simulink model "VMC_LateralTrajectoryPlanningControllerV04"  (R2018b)
settings: Solver=FixedStepDiscrete  StartTime=0.0  StopTime=10  FixedStep=0.02  RelTol=1e-3
values from neighbouring files (symbols this model uses):
  D_d_end = 0    [TRP_parameters.m]
  P_optimizer_interations = 5.0    (= 5)    [TRP_parameters.m]
  P_TRP_Lat_dT = 0.02    [TRP_parameters.m]
  P_Vehicle_width = 1.8    [TRP_parameters.m]
  P_vVeh_min_TrajCalc = 5.0    (= 5)    [TRP_parameters.m]
libraries: simulink x1
(part 2 of 2)

== matlab function VMC_LateralTrajectoryPlanningControllerV04/VMC_LateralTrajectoryPlanningController/LatTRP_GenerateTraj/MATLAB Function ==
  data: vVeh input; SafetyDistance input; B_StartOptimization input; B_StopOptimization input; d_start input; d_d_start input; d_dd_start input; d_ddd_start_K1 input; t_max_in input; t_min_in input; k_j input; k_v input; k_t input; k_cy input; k_j_y_constraint input; k_a_y_constraint input; k_overshoot input; k_jy_change_sq input; j_y_constraint input; a_y_constraint input; d_overshootAllowed input; d_left_yellow input; d_right_yellow input; d_end input; P_vVeh_min_TrajCalc parameter; P_optimizer_interations parameter; P_TRP_Lat_dT parameter; P_Vehicle_width parameter; d0 output; d1 output; d2 output; d3 output; d4 output; d5 output; s_end_traj output; c2 input; t_Winner output
function [d0, d1, d2, d3, d4, d5, s_end_traj, t_Winner] = fcn(vVeh,SafetyDistance,B_StartOptimization,B_StopOptimization,d_start,d_d_start,d_dd_start,d_ddd_start_K1,t_max_in,...
                                              t_min_in,k_j,k_v,k_t,k_cy,k_j_y_constraint,k_a_y_constraint,k_overshoot,k_jy_change_sq,j_y_constraint,a_y_constraint,...
                                              d_overshootAllowed, d_left_yellow,d_right_yellow,d_end,P_vVeh_min_TrajCalc,...
                                              P_optimizer_interations,P_TRP_Lat_dT,P_Vehicle_width, c2)
D_dT = P_TRP_Lat_dT;

persistent d0_K1;
persistent d1_K1;
persistent d2_K1;
persistent d3_K1;
persistent d4_K1;
persistent d5_K1;
persistent t_min_K1
persistent t_max_K1
persistent alreadyCalculated
persistent t
persistent d3_opt
persistent d4_opt
persistent d5_opt
persistent a_y_violation
persistent j_y_violation
persistent jerk_sq_int
persistent jy_change_sq
persistent vel_sq_int
persistent cost
persistent violation_sq_left_yellow_int
persistent violation_sq_right_yellow_int
persistent d_overshoot_violation
persistent s_end_traj_
persistent winner

if isempty(d0_K1)
    d0_K1 = 0;
    d1_K1 = 0;
    d2_K1 = 0;
    d3_K1 = 0;
    d4_K1 = 0;
    d5_K1 = 0;
    t_min_K1 = 0;
    t_max_K1 = 0;
    alreadyCalculated = false(5,1);
    t = zeros(5,1);
    d3_opt = zeros(5,1);
    d4_opt = zeros(5,1);
    d5_opt = zeros(5,1);
    a_y_violation = zeros(5,1);
    j_y_violation = zeros(5,1);
    jerk_sq_int = zeros(5,1);
    jy_change_sq = zeros(5,1);
    vel_sq_int = zeros(5,1);
    cost = zeros(5,1);
    violation_sq_left_yellow_int = zeros(5,1);
    violation_sq_right_yellow_int = zeros(5,1);
    d_overshoot_violation = zeros(5,1);
    s_end_traj_ = 0;
    winner = 1;
end

% fisrt three coefficients are independent of the trajecotry length
d0_opt = d_start;
d1_opt = d_d_start;
d1_opt_p2 = d1_opt * d1_opt;
d2_opt = 0.5 * d_dd_start;
d2_opt_p2 = d2_opt * d2_opt;

% start values for the duration for the optimization
% if B_startoptimization flag is true, new trajectory optimization starts
% get the initial trajectory length limits from input arguments;

if B_StartOptimization == true
    t_min = t_min_in;
    t_max = t_max_in;
    
    alreadyCalculated(1) = false;
    alreadyCalculated(2) = false;
    alreadyCalculated(3) = false;
    alreadyCalculated(4) = false;
    alreadyCalculated(5) = false;
% otherwise, set the trajectory length limits according to the best
% trajectory from previous cycle
else
    t_min = t_min_K1;
    t_max = t_max_K1;
end

% limit velocity to prevent short and vary dynamic trajecotry at low
% velocity
vVeh_lim = vVeh;
vVeh_lim = max(vVeh_lim,P_vVeh_min_TrajCalc);
vVeh_lim_p2 = vVeh_lim * vVeh_lim;
vVeh_lim_p4 = vVeh_lim_p2 * vVeh_lim_p2;
vVeh_lim_p6 = vVeh_lim_p4 * vVeh_lim_p2;

% if both B_startoptimization B_stopoptimization flags are true
% it indicates all the optimization interations will be done in one
% calculation cycle

if B_StartOptimization == true && B_StopOptimization == true
    
    OptimizerInterations = P_optimizer_interations;
    % otherwise only one optimization interation will run during each
    % calculation cycle
else
    OptimizerInterations = 1;
end

for index = 1:OptimizerInterations
    % divide interval
    delta_t = (t_max - t_min) / 4;
    t(1) = t_min;
    t(2) = t_min + delta_t;
    t(3) = t_min + 2 * delta_t;
    t(4) = t_min + 3 * delta_t;
    t(5) = t_max;
    
    for i = 1:5
        i_lim = min(i,5);
        % only calculate and evaluate the trajectory if it has not already
        % been calculated and evaluated in the previous iteration
        % short and dynamic trajectories at low speed
        if ~alreadyCalculated(i_lim)
            s_end = t(i_lim) * vVeh_lim;
            s_end_p2 = s_end * s_end;
            s_end_p3 = s_end_p2 * s_end;
            s_end_p4 = s_end_p3 * s_end;
            s_end_p5 = s_end_p4 * s_end;
            s_end_p6 = s_end_p5 * s_end;
            s_end_p7 = s_end_p6 * s_end;
            s_end_p8 = s_end_p7 * s_end;
            s_end_p9 = s_end_p8 * s_end;
            
             % calculate remaining coefficient;
            d3_opt(i_lim) = -(3 * d_dd_start * s_end_p2 + 12  * d_d_start * s_end - 20 * d_end + 20 * d_start) / (2 * s_end_p3);
            d3_opt_p2 = d3_opt(i_lim) * d3_opt(i_lim);
            d4_opt(i_lim) = (3 * d_dd_start * s_end_p2 + 16 * d_d_start * s_end - 30 * d_end + 30 * d_start) / (2 * s_end_p4);
            d4_opt_p2 = d4_opt(i_lim) * d4_opt(i_lim);
            d5_opt(i_lim) = -(d_dd_start * s_end_p2 + 6 * d_d_start * s_end - 12 * d_end + 12 * d_start) / (2 * s_end_p5);
            d5_opt_p2 = d5_opt(i_lim) * d5_opt(i_lim);
            
            % calculate points on trajectory with max kappa if d5 is not
            % too close to 0 (division by 0)
            
            if abs(d5_opt(i_lim)) > 1e-20
                s_kappa_max_temp = (2 * d4_opt(i_lim)) / (10 * d5_opt(i_lim)) * (2 * d4_opt(i_lim)) / (10 * d5_opt(i_lim)) - d3_opt(i_lim) / (10 * d5_opt(i_lim));
                s_kappa_max_temp = sqrt(s_kappa_max_temp);
                s_kappa_max_1 = -(2 * d4_opt(i_lim)) / (10 * d5_opt(i_lim)) - s_kappa_max_temp;
                s_kappa_max_1 = max(0,s_kappa_max_1);
                s_kappa_max_1 = min(s_kappa_max_1,s_end);
                s_kappa_max_2 = -(2 * d4_opt(i_lim)) / (10 * d5_opt(i_lim)) + s_kappa_max_temp;
                s_kappa_max_2 = max(s_kappa_max_2,0);
                s_kappa_max_2 = min(s_kappa_max_2,s_end);
                
                
                s_kappa_max_1_p2 = s_kappa_max_1 * s_kappa_max_1;
                s_kappa_max_1_p3 = s_kappa_max_1_p2 * s_kappa_max_1;
                
                s_kappa_max_2_p2 = s_kappa_max_2 * s_kappa_max_2;
                s_kappa_max_2_p3 = s_kappa_max_2_p2 * s_kappa_max_2;
            else
                % if d5 is too close to 0 then set the position to -1 
                % this will lead to neglecting the maximum lateral
                % acceleratio in the cost function
                % s_kappa_max_temp = -1;
                s_kappa_max_1 = -1;
                s_kappa_max_2 = -1;
                
                s_kappa_max_1_p2 = -1;
                s_kappa_max_1_p3 = -1;
                
                s_kappa_max_2_p2 = -1;
                s_kappa_max_2_p3 = -1;
                
                 % Idea: if d5 is chose to 0,then calculate max lateral acceleration with polynomial of degree 4 if possible
            end
            
            % calculate max lateral acceleration under the assumption of constant curvature and vehicle velocity. but only if the
            % point at a relevant position(>= 0 and <= planned length s_end)
            
            if (s_kappa_max_1 >= 0 && s_kappa_max_1 <= s_end)
                a_y_1_abs = vVeh * vVeh * c2 + vVeh * vVeh * (2 * d2_opt + 6 * d3_opt(i_lim) * s_kappa_max_1 + 12 * d4_opt(i_lim) * s_kappa_max_1_p2 + 20 * d5_opt(i_lim) * s_kappa_max_1_p3);
                a_y_1_abs = abs(a_y_1_abs);
            else
                a_y_1_abs = 0;
            end
            
            if (s_kappa_max_2 >= 0 && s_kappa_max_2 <= s_end)
                a_y_2_abs = vVeh * vVeh * c2 + vVeh * vVeh * (2 * d2_opt + 6 * d3_opt(i_lim) * s_kappa_max_2 + 12 * d4_opt(i_lim) * s_kappa_max_2_p2 + 20 * d5_opt(i_lim) * s_kappa_max_2_p3);
                a_y_2_abs = abs(a_y_2_abs);
            else
                a_y_2_abs = 0;
            end
            % find maximum acceleration value
            % start and end is not considered because they are both boundary conditions
            a_abs_max = a_y_1_abs;
            a_abs_max = max(a_abs_max,a_y_2_abs);
            a_y_violation(i_lim) = a_abs_max - a_y_constraint;
            a_y_violation(i_lim) = max(a_y_violation(i_lim),0);
            
             % find max jerk in trajectory under the assumption: the
            % reference line has no jerk itself (constant curvature)
            % find position of extremum and calculate the jerk at this position
            if abs(d5_opt(i_lim)) > 1e-20
                s_jerk_max = -24 * d4_opt(i_lim) / (120 * d5_opt(i_lim));
                
                % limit position to trajectory length
                s_jerk_max = max(s_jerk_max,0);
                s_jerk_max = min(s_jerk_max,s_end);
                
                % calculate lateral jerk at extremum
                j_y_l_abs = vVeh * vVeh * vVeh * (6 * d3_opt(i_lim) + 24 * d4_opt(i_lim) * s_jerk_max + 60 * d5_opt(i_lim) * s_jerk_max * s_jerk_max);
                j_y_l_abs = abs(j_y_l_abs);
            else
                % if d5 is 0 then the jerk is linear, therefore the
                % absolute maximum of the lateral jerk of the trajectory
                % has to occur at the position 0 and s_end (they are
                % covered by j_y_2_abs and j_y_3_abs)
                % s_jerk_max = 0;
                j_y_l_abs = 0;
            end
            % calculate lateral jerk at the start and at the end of the
            % trajectory
            j_y_2_abs = vVeh * vVeh * vVeh * (6 * d3_opt(i_lim) + 24 * d4_opt(i_lim) * s_end + 60 * d5_opt(i_lim) * s_end_p2);
            j_y_2_abs = abs(j_y_2_abs);
            j_y_3_abs = vVeh * vVeh * vVeh * 6 * d3_opt(i_lim);
            j_y_3_abs = abs(j_y_3_abs);
            j_abs_max = j_y_l_abs;
            j_abs_max = max(j_abs_max,j_y_2_abs);
            j_abs_max = max(j_abs_max,j_y_3_abs);
            
            j_y_violation(i_lim) = j_abs_max - j_y_constraint;
            j_y_violation(i_lim) = max(j_y_violation(i_lim),0);
            
             % calculate the integral of jerk squared
            jerk_sq_int(i_lim) = (12 * s_end * vVeh_lim_p6 * (3 * d3_opt_p2 + 12 * d3_opt(i_lim) * d4_opt(i_lim) * s_end + 20 * d3_opt(i_lim) * d5_opt(i_lim) * s_end_p2 + 16 * d4_opt_p2 * s_end_p2 + 60 * d4_opt(i_lim) * d5_opt(i_lim) * s_end_p3 + 60 * d5_opt_p2 * s_end_p4)) / vVeh_lim;
            
            % calculate the change in lateral jerk squared at the beginning
            % of the trajectory(compared to the lateral jerk at the
            % beginning of the last trajectory)
            jy_change_sq(i_lim) = vVeh * vVeh * vVeh * (6 * d3_opt(i_lim) - d_ddd_start_K1);
            jy_change_sq(i_lim) = jy_change_sq(i_lim) * jy_change_sq(i_lim);
            
            % calculate the integral of acceleration squared
            % accel_sq_int = (4 *d2_p2 * s_end * vVeh_lim_p4 + (s_end_p3 * vVeh_lim_p4 *(36 * d3_opt_p2 + 48 * d2 *d4_opt(i_lim))/3 +  (s_end_p5 * vVeh_lim_p4 * (144 * d4_opt_p2 + 240 * d3_opt(i_lim) * d5_opt(i_lim)) / 5 + (s_end_p4 * vVeh_lim_p4 * (80 * d2 * d5_opt(i_lim) + 144 * d4_opt(i_lim) * d4_opt(i_lim)) / 4 + (400 * d5_opt_p2 * s_end_p7 * vVeh_lim_p4) / 7 + 12 * d2 * d3_opt(i_lim) * s_end_p2 * vVeh_lim_p4 + 80 * d4_opt(i_lim) * d5_opt(i_lim) * s_end_p6 * vVeh_lim_p4) / vVeh_lim;
            
            % calculate the integral of velocity squared
            vel_sq_int(i_lim) = (d1_opt_p2 * s_end * vVeh_lim_p2 + (s_end_p3 * vVeh_lim_p2 * (4 * d2_opt_p2 + 6 * d1_opt * d3_opt(i_lim))) / 3 + (s_end_p7 * vVeh_lim_p2 * (16 * d4_opt_p2 + 30 * d3_opt(i_lim) * d5_opt(i_lim))) / 7 + (s_end_p4 * vVeh_lim_p2 * (8 * d1_opt * d4_opt(i_lim) + 12 * d2_opt * d3_opt(i_lim))) / 4 + (s_end_p6 * vVeh_lim_p2 * (20 * d2_opt * d5_opt(i_lim)+ 24 * d3_opt(i_lim) * d4_opt(i_lim))) / 6 + (25 * d5_opt_p2 * s_end_p9 * vVeh_lim_p2) / 9 + (s_end_p5 * vVeh_lim_p2 * (9 * d3_opt_p2 + 10 * d1_opt * d5_opt(i_lim) + 16 * d2_opt * d4_opt(i_lim))) / 5 + 2 * d1_opt * d2_opt * s_end_p2 * vVeh_lim_p2 + 5 * d4_opt(i_lim) * d5_opt(i_lim) * s_end_p8 * vVeh_lim_p2) / vVeh_lim;
            
             % calculate the space of violation of left yellow corridor border
            [violationAreaLeft,violationAreaRight] = LatCorridorViolationCheck(P_Vehicle_width,SafetyDistance,d0_opt,d1_opt,d2_opt,d3_opt(i_lim),d4_opt(i_lim),d5_opt(i_lim),s_end,d_left_yellow,d_right_yellow,vVeh_lim);
           %%
            violation_sq_left_yellow_int(i_lim) = violationAreaLeft;
            violation_sq_right_yellow_int(i_lim) = violationAreaRight;

            % check if trajectory is overshooting
           %%
            d_overshoot_abs = LatCalcTrajOvershoot(d0_opt,d1_opt,d2_opt,d3_opt(i_lim),d4_opt(i_lim),d5_opt(i_lim),s_end);
           %%
            d_overshoot_violation(i_lim) = d_overshoot_abs - d_overshootAllowed;
            d_overshoot_violation(i_lim) = max(d_overshoot_violation(i_lim),0);
             % calculate cost function with weighted sum of all costs
            cost(i_lim) = k_j * jerk_sq_int(i_lim) + k_v * vel_sq_int(i_lim) + k_cy * (violation_sq_left_yellow_int(i_lim) + violation_sq_right_yellow_int(i_lim)) + k_t * t(i_lim) + k_a_y_constraint * a_y_violation(i_lim) + k_j_y_constraint * j_y_violation(i_lim) + k_overshoot * d_overshoot_violation(i_lim) + k_jy_change_sq * jy_change_sq(i_lim);
        else
            % this trajectory has already been calculated and evaluated in
            % the previous iteration
        end
        
         % check for the best result
        if (i > 1)
            if cost(i_lim) < cost(winner)
                winner = i_lim;
            end
        else
            winner = 1;
        end     
    end
    
    % set duration limits for next optimization
    if winner == 1
        t_min = t(1);
        t_max = t(2);
        
        % the trajectories 0 from the current iteration will also be
        % trajecotry 0 in the next interation
        alreadyCalculated(1) = true;
        
        % this array elements are already filled correctly, ao no shifting
        % necesaary
        % the trajectories 1,2 and 3 will have to be calculated and evalted
        % in the next interation
        alreadyCalculated(2) = false;
        alreadyCalculated(3) = false;
        alreadyCalculated(4) = false;
        
        % the trajectory 1 of the current iteration will become trajectory
        % 4 in the next iteration
        alreadyCalculated(5) = true;
        d3_opt(5) = d3_opt(2);
        d4_opt(5) = d4_opt(2);
        d5_opt(5) = d5_opt(2);
        cost(5) = cost(2);
        jerk_sq_int(5) = jerk_sq_int(2);
        vel_sq_int(5) = vel_sq_int(2);
        violation_sq_left_yellow_int(5) = violation_sq_left_yellow_int(2);
        violation_sq_right_yellow_int(5) = violation_sq_right_yellow_int(2);
        a_y_violation(5) = a_y_violation(2);
        j_y_violation(5) = j_y_violation(2);
        jy_change_sq(5) = jy_change_sq(2);
        % no setting of already calculated t values because this will
        % calculated in the next cycle from t_min and t_max
    elseif winner == 5
        t_min = t(4);
        t_max = t(5);
        
        % the trajectory 3 of the current iteration will be trajectory 0 in
        % the next iteration
        alreadyCalculated(1) = true;
        d3_opt(1) = d3_opt(4);
        d4_opt(1) = d4_opt(4);
        d5_opt(1) = d5_opt(4);
        cost(1) = cost(4);
        jerk_sq_int(1) = jerk_sq_int(4);
        vel_sq_int(1) = vel_sq_int(4);
        violation_sq_left_yellow_int(1) = violation_sq_left_yellow_int(4);
        violation_sq_right_yellow_int(1) = violation_sq_right_yellow_int(4);
        a_y_violation(1) = a_y_violation(4);
        j_y_violation(1) = j_y_violation(4);
        d_overshoot_violation(1) = d_overshoot_violation(4);
        jy_change_sq(1) = jy_change_sq(4);
        
        % no setting of the already calculated t values because this will
        % be calculated in the next cycle from t_min and t_max
        alreadyCalculated(2) = false;
        alreadyCalculated(3) = false;
        alreadyCalculated(4) = false;
        
        % the trajectory 4 of the current iteration will also be trajectory
        % 4 in the next iteration
        alreadyCalculated(5) = true;
        % this array elements are already filled correctly, so no shifting
        % necessary
    else
        t_min = t(winner - 1);
        t_max = t(winner + 1);
        
        % the trajectory winner - 1 of the current iteration will be
        % trajectory 0 in the next iteration
        alreadyCalculated(1) = true;
        d3_opt(1) = d3_opt(winner - 1);
        d4_opt(1) = d4_opt(winner - 1);
        d5_opt(1) = d5_opt(winner - 1);
        cost(1) = cost(winner - 1);
        jerk_sq_int(1) = jerk_sq_int(winner - 1);
        vel_sq_int(1) = vel_sq_int(winner - 1);
        violation_sq_left_yellow_int(1) = violation_sq_left_yellow_int(winner - 1);
        violation_sq_right_yellow_int(1) = violation_sq_right_yellow_int(winner - 1);
        a_y_violation(1) = a_y_violation(winner - 1);
        j_y_violation(1) = j_y_violation(winner - 1);
        d_overshoot_violation(1) = d_overshoot_violation(winner - 1);
        jy_change_sq(1) = jy_change_sq(winner - 1);
        % no setting of the already calculated t values because this will
        % be calculated in the next cycle from t_min and t_max 
        alreadyCalculated(2) = false;
        alreadyCalculated(3) = false;
        alreadyCalculated(4) = false;
        
        % the trajectory winner + 1 of the current iteration will become
        % trajectory 4 in the next iteration
        alreadyCalculated(5) = true;
        d3_opt(5) = d3_opt(winner + 1);
        d4_opt(5) = d4_opt(winner + 1);
        d5_opt(5) = d5_opt(winner + 1);
        cost(5) = cost(winner + 1);
        jerk_sq_int(5) = jerk_sq_int(winner + 1);
        vel_sq_int(5) = vel_sq_int(winner + 1);
        violation_sq_left_yellow_int(5) = violation_sq_left_yellow_int(winner + 1);
        violation_sq_right_yellow_int(5) = violation_sq_right_yellow_int(winner + 1);
        a_y_violation(5) = a_y_violation(winner + 1);
        j_y_violation(5) = j_y_violation(winner + 1);
        d_overshoot_violation(5) = d_overshoot_violation(winner + 1);
        jy_change_sq(5) = jy_change_sq(winner + 1);
        % no setting of the already calculated t values because this will
        % be calculated in the next cycle from t_min and t_max
    end

end

% if B_StopOptimization flag is true, the optimization is finished the
% trajectory with lowest cost is the final optimal one
if B_StopOptimization == true
    d0 = d0_opt;
    d1 = d1_opt;
    d2 = d2_opt;
    d3 = d3_opt(winner);
    d4 = d4_opt(winner);
    d5 = d5_opt(winner);
    
    % set trajectory length
    s_end_traj_ = t(winner) * vVeh_lim;
else
% % otherwise, the optimization is not yet finished, in that case the optimal
% % trajectory of the last full optimization cycle is used just do the
% % coefficients compensation, for start boundary conditions calculation in
% % next cycle
    delta_s = vVeh * D_dT;
    delta_s_p2 = delta_s * delta_s;
    delta_s_p3 = delta_s_p2 * delta_s;
    delta_s_p4 = delta_s_p3 * delta_s;
    delta_s_p5 = delta_s_p4 * delta_s;
    
    d0 = d0_K1 + d1_K1 * delta_s + d2_K1 * delta_s_p2 + d3_K1 * delta_s_p3 + d4_K1 * delta_s_p4 + d5_K1 * delta_s_p5;
    d1 = d1_K1 + 2 * d2_K1 * delta_s + 3 * d3_K1 * delta_s_p2 + 4 * d4_K1 * delta_s_p3 + 5 * d5_K1 *delta_s_p4;
    d2 = d2_K1 + 3 * d3_K1 * delta_s + 6 * d4_K1 * delta_s_p2 + 10 * d5_K1 * delta_s_p3;
    d3 = d3_K1 + 4 * d4_K1 * delta_s + 10 * d5_K1 * delta_s_p2;
    d4 = d4_K1 + 5 * d5_K1 * delta_s;
    d5 = d5_K1;
    
    % set trajectory length
    s_end_traj_ = s_end_traj_ - delta_s;
end

d0_K1 = d0;
d1_K1 = d1;
d2_K1 = d2;
d3_K1 = d3;
d4_K1 = d4;
d5_K1 = d5;

t_min_K1 = t_min;
t_max_K1 = t_max;

s_end_traj = s_end_traj_;  
t_Winner = t(winner);

%%
% dist_x = d0 : 100;
% dist_y = d0 + d1 * dist_x + d2 * dist_x.^2 + d3_opt * dist_x.^3 + d4_opt * dist_x.^4 + d5_opt * dist_x.^5;
% handles = plot(dist_x, dist_y, 'r');
% pause (0.03);
% delete handles;
%%

function [violationAreaLeft,violationAreaRight] = LatCorridorViolationCheck(vehicleWidth,safetyDistance,d0,d1,d2,d3,d4,d5,s_end,d_StaticCorridorLeft,d_StaticCorridorRight,vVeh)
P_k_cy_vy_CurX = [-0.2 -0.1 0 0.1 0.2];
P_k_cy_vy_CurY = [0.01 0.01 0.01 0.7 1.0];
D_nPtsViolationCheck = 20;
D_sMaxViolationCheck = 100;
violationAreaLeft = 0;
violationAreaRight = 0;
nEvals = D_nPtsViolationCheck;
deltaS = D_sMaxViolationCheck/nEvals;
for j = 1:D_nPtsViolationCheck
    iFloat = j;
    s = iFloat * deltaS;
    s_p2 = s * s;
    s_p3 = s * s_p2;
    s_p4 = s * s_p3;
    s_p5 = s * s_p4;
    
    if s <= s_end
        d = d0 + d1 * s + d2 * s_p2 + d3 * s_p3 + d4 * s_p4 + d5 * s_p5;
        d_left = d + 0.5 * vehicleWidth + safetyDistance;
        d_right = d - 0.5 * vehicleWidth - safetyDistance;
        
        % approximation of planned lateral velocity by first derivative of trajectory multiplied by vehicle
        % longitudinal velocity 
        vy = vVeh * (d1 + 2 * d2 * s + 3 * d3 * s_p2 + 4 * d4 * s_p3 + 5 * d5 * s_p4);
        % check violation of left corridor border
        if d_left > d_StaticCorridorLeft
            k_cy_vy = lookforchart(P_k_cy_vy_CurX,P_k_cy_vy_CurY,vy);
            violationAreaLeft = violationAreaLeft + k_cy_vy * (d_left - d_StaticCorridorLeft) * deltaS;
        else
            % no violation of the left corridor border
        end
        % check violation of right corridor border
        if d_right < d_StaticCorridorRight
            k_cy_vy = lookforchart(P_k_cy_vy_CurX,P_k_cy_vy_CurY,-vy);
            violationAreaRight = violationAreaRight + k_cy_vy * (d_StaticCorridorRight - d_right) * deltaS;
        else
            % no violation of the right corridor border
        end
    else
        %vehicle already is on the reference line (middle of the blue
        %static corridor) --> no additional violation
        break;
    end   
end
end

function d_overshoot_abs= LatCalcTrajOvershoot(d0,d1,d2,d3,d4,d5,s_end)
% The trajectory describes the lateral offset to the reference line. form as
% d(s) = d0 + d1 * s + d2 * s^2 + d3 * s^3 + d4 * s^4 + d5 * s^5
% dd(s) = d1 + 2 * d2 * s + 3 * d3 * s^2 + 4 * d4 * s^3 + 5 * d5 * s^4
% This class is to calculate the absolute overshoot distance for its cost in the optimization weight 
% During emergency maneuvers, it is common that the planner would try to correct the current yaw rate quickly
% It will lead to some overshoot path planning issues. For the current jerk based optimization ad comfort requirement, the overshoot planning should be avoided in the TRP
% To ensure if the current planning has a overshoot, the roots of dd(s) = 0 have to be calculated to find the extrem values
% since d(s_end) = 0 ,dd(s_end) = 0 ddd(s_end) = 0 are considered as initial condition
% the dd(s) function can be simplified as dd(s) = (s - s_end)^2 * (a * s^2 + b * s + c), refer FD for more explanation 
% Expend the equation and align with the corresponded part in the original dd(s) to calculate the coefficient
a = 5 * d5;
b = 4 * d4 + 2 * a * s_end;
c = 3 * d3 + 2 * b * s_end - a * s_end * s_end;
% reinit overshoot value each time
d_overshoot_abs = 0;
% check if a,b are equal to 0
if a == 0
    TCH_IsEqual_a = true;
else
    TCH_IsEqual_a = false;
end

if b == 0
   TCH_IsEqual_b = true;
else
   TCH_IsEqual_b = false;
end
% To calculate the maximum overshoot
if TCH_IsEqual_a && TCH_IsEqual_b
    % no overshoot
elseif TCH_IsEqual_a && ~TCH_IsEqual_b
    % linear equation, only one root
    s = - c / b;
    if s > 0 && s < s_end
        s_p2 = s * s;
        s_p3 = s_p2 * s;
        s_p4 = s_p3 * s;
        s_p5 = s_p4 * s;
        d = d0 + d1 * s + d2 * s_p2 + d3 * s_p3 + d4 * s_p4 + d5 * s_p5;
        if (d0 * d < 0)
            d_overshoot_abs = abs(d);
        else
        end
    else
    end
else
    delta = b * b - 4 * a * c;
    if delta < 0
        % no real root no overshoot
    else
        %to find two roots
        delta_sqrt = sqrt(delta);
        s_1 = (-b + delta_sqrt) / (2 * a);
        s_2 = (-b - delta_sqrt) / (2 * a);
        % to ensure roots are within s0 and s_end
        if s_1 > 0 && s_1 < s_end
            s = s_1;
            s_p2 = s * s;
            s_p3 = s_p2 * s;
            s_p4 = s_p3 * s;
            s_p5 = s_p4 * s;
            d = d0 + d1 * s + d2 * s_p2 + d3 * s_p3 + d4 * s_p4 + d5 * s_p5;
            if d0 * d < 0
                d_overshoot_abs = abs(d);
            else
            end
        else
        end
        
        if s_2 > 0 && s_2 < s_end
            s = s_2;
            s_p2 = s * s;
            s_p3 = s_p2 * s;
            s_p4 = s_p3 * s;
            s_p5 = s_p4 * s;
            d = d0 + d1 * s + d2 * s_p2 + d3 * s_p3 + d4 * s_p4 + d5 * s_p5;
            if d0 * d < 0
                d_overshoot_abs = max(d_overshoot_abs,abs(d));
            else
            end
        else
        end
    end
end
end
end

== matlab function VMC_LateralTrajectoryPlanningControllerV04/VMC_LateralTrajectoryPlanningController/VMC_TRPLat_TargetPathPrep/MATLAB Function ==
  data: c0 input; pp_c00 output; c1 input; c2 input; c3 input; d0 input; d1 input; d2 input; d3 input; pp_c01 output; pp_c02 output; pp_c03 output; pp_c04 output; pp_c05 output; d4 input; d5 input
function [pp_c00,pp_c01,pp_c02,pp_c03,pp_c04,pp_c05] = fcn(c0,c1,c2,c3,d0,d1,d2,d3,d4,d5)

% target path and derivatives wer x at zero in current "target path frame"
% remark: for small angels, the combination of frenet-path and reference
% line is obtained by simply adding the coefficients of the polynomials,
% which is valid when assuming that the arc length of the target path is
% equal to the projection of the target path along the y-axis of the
% vechile corrdinate frame 

% piecewise polynomial 1
% pp_c00 = c0 + d0;
% pp_c01 = c1 + d1;
% pp_c02 = c2 + 2 * d2;
% pp_c03 = c3 + 6 * d3;
% pp_c04 = 24 * d4;
% pp_c05 = 120 * d5;

% piecewise polynomial 2
% pp_c10 = c0;
% pp_c11 = c1;
% pp_c12 = c2;
% pp_c13 = c3;

% piecewise polynomial 1
pp_c00 = c0 + d0;
pp_c01 = c1 + d1;
pp_c02 = c2 + d2;
pp_c03 = c3 + d3;
pp_c04 = d4;
pp_c05 = d5;
